simulink model "FinalModel"  (R2022a)
settings: Solver=VariableStepAuto  StartTime=0.0  StopTime=2  RelTol=1e-3
libraries: visionsources x2
settings Model: Creator=RAJSEKHAR  LastModifiedBy=RAJSEKHAR
settings ConfigComp: CovEnable=on  RecordCoverage=on  CovModelRefEnable=on

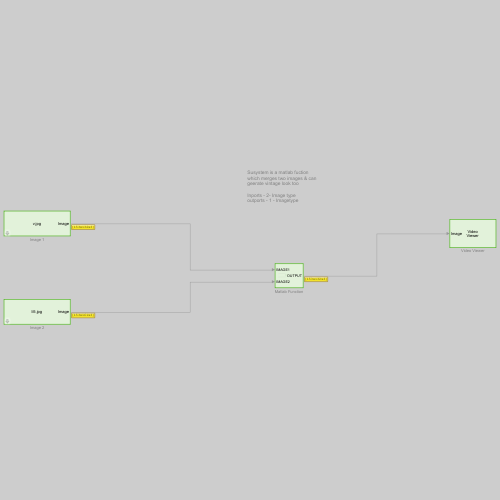
[thumbnail: Simulink's stored preview of the top-level diagram]
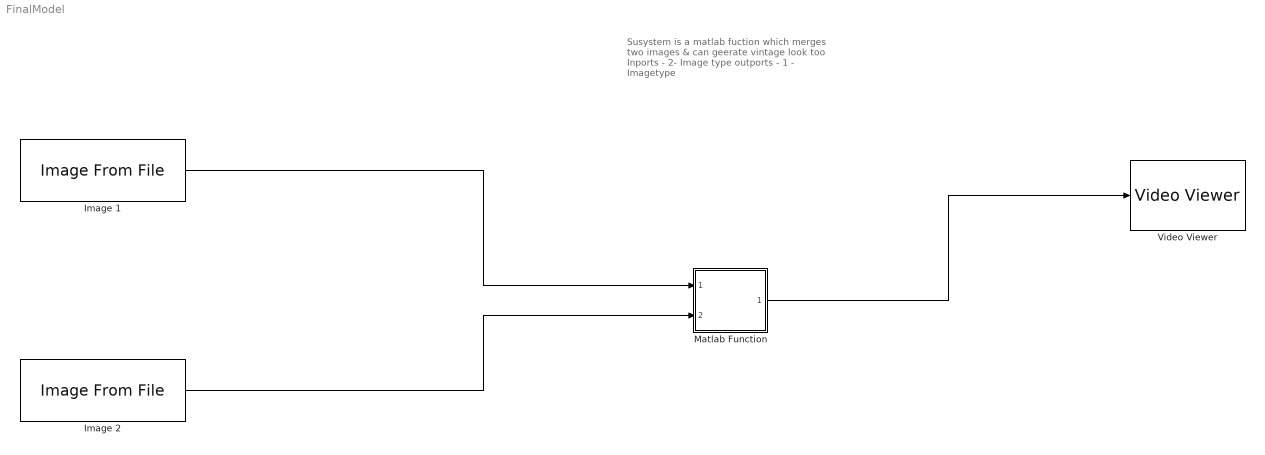
== system FinalModel ==
  note: Susystem is a matlab fuction
      | which merges two images & can geerate vintage look too
      |
      | Inports - 2- Image type
      | outports - 1 - Imagetype
  Image 1 : visionsources/Image From File  Tag=vipblks_nd  FileName=D:\Users\RAJSEKHAR\Downloads\v.jpg  Ts=inf  imagePorts=One multidimensional signal  OutPortLabels=R|G|B  ImageDataType=Inherit from input image  sdImageDataType=uint(8)  Signed=on  WordLength=16  FractionLengthMode=User-defined  FractionLength=15
  Image 2 : visionsources/Image From File  Tag=vipblks_nd  FileName=D:\Users\RAJSEKHAR\Downloads\li5.jpg  Ts=inf  imagePorts=One multidimensional signal  OutPortLabels=R|G|B  ImageDataType=Inherit from input image  sdImageDataType=uint(8)  Signed=on  WordLength=16  FractionLengthMode=User-defined  FractionLength=15
  Matlab Function : Subsystem
  Video Viewer : VideoViewer  FigPos=[1376 392 357 191]
  wires:
  Matlab Function/1(OUTPUT) -> Video Viewer/1
  Image 1/1 -> Matlab Function/1(IMAGE1)
  Image 2/1 -> Matlab Function/2(IMAGE2)

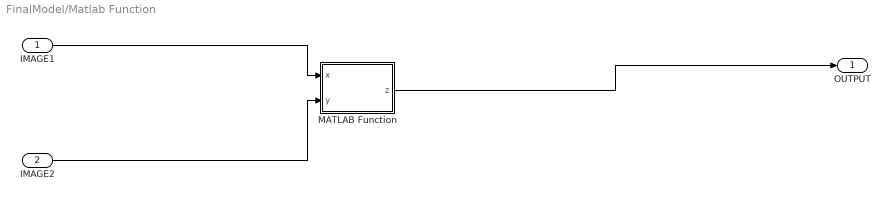
== system FinalModel/Matlab Function ==
  IMAGE1 : Inport
  IMAGE2 : Inport  Port=2
  MATLAB Function : MATLAB Function  TreatAsAtomicUnit=on
  OUTPUT : Outport
  wires:
  IMAGE2/1 -> MATLAB Function/2(y)
  IMAGE1/1 -> MATLAB Function/1(x)
  MATLAB Function/1(z) -> OUTPUT/1

== matlab function FinalModel/Matlab Function/MATLAB Function ==
  data: x input; z output; y input
function z = fcn(x, y)

%  clc
% clear
% close all
% warning off;
%  x=imread('D:\Users\RAJSEKHAR\Downloads\red2.jpg');
%  y=imread('D:\Users\RAJSEKHAR\Downloads\rect2.jpg');
g=size(x);
y=imresize(y,[g(1),g(2)]);
figure;
z=x-y;
pause(5);
